simulink model "tractioncontrol_rmse22_nobrakes"  (R2022a)
settings: Solver=VariableStepAuto  StartTime=0.0  StopTime=48  RelTol=1e-3
values from neighbouring files (symbols this model uses):
  A = 1.08    [test_script.m]
  Cd = 1.02    [test_script.m]
  g = 9.81    [test_script.m]
  gr = 47/13    (= 3.61538461538)    [test_script.m]
  h_cg = .259    (= 0.259)    [test_script.m]
  h_d = h_cg    (= 0.259)    [test_script.m]
  J = 0.27    [test_script.m]
  m = 297    [test_script.m]
  r = 0.5588    [test_script.m]
  rho = 1.162    [test_script.m]
  wb = 1.53    [test_script.m]
undefined symbols (not defined in the file or in its folder): batt_Vnom, Conv_eff, front_wb, initial_SOC, motor_eff, normalized_voltage, Qmax, SOC
libraries: simulink x2, slpidlib x1
settings Model: Creator=Asus  LastModifiedBy=sahil
settings SolverCC: AlgebraicLoopSolver=TrustRegion
settings RTWCC: DLArmComputeVersion=19.05

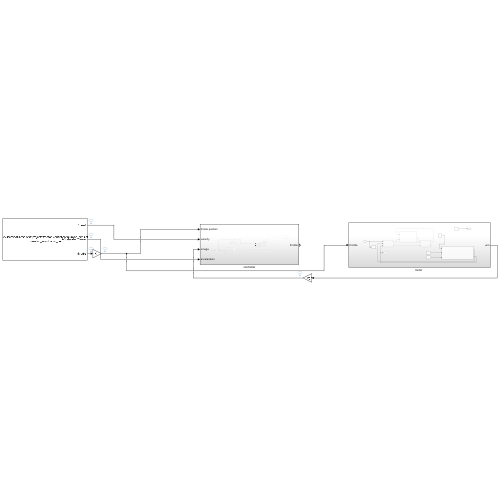
[thumbnail: Simulink's stored preview of the top-level diagram]
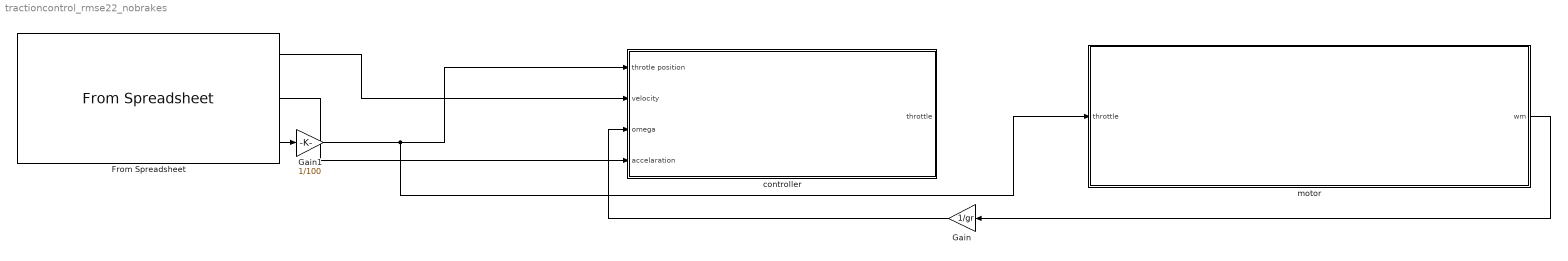
== system tractioncontrol_rmse22_nobrakes ==
  From Spreadsheet : FromSpreadsheet  FileName=C:\Users\sahil\rms stuff\projects\traction control\optimumlap_simulations\simulation_resultsssss_aaa.csv  SheetName=simulation_resultsssss_aaa
  Gain : Gain  Gain=1/gr
  Gain1 : Gain  Gain=1/100
  controller : Subsystem
  "motor  " : Subsystem
  wires:
  From Spreadsheet/3 -> Gain1/1
  "motor  "/1(wm) -> Gain/1
  Gain/1 -> controller/3(omega)
  From Spreadsheet/1 -> controller/2(velocity)
  From Spreadsheet/2 -> controller/4(accelaration)
  Gain1/1 -> "motor  "/1(throttle), controller/1(throtle position)

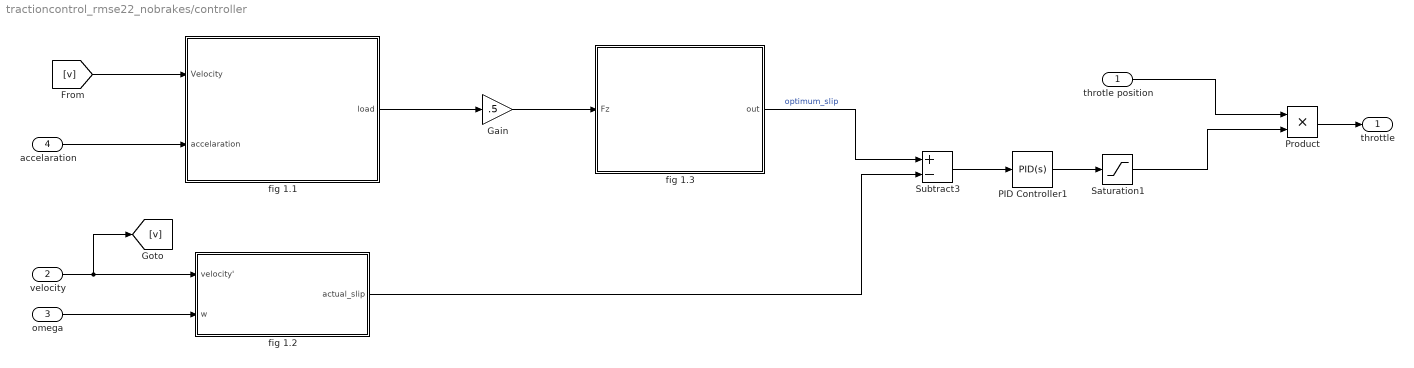
== system tractioncontrol_rmse22_nobrakes/controller ==
  throtle position : Inport
  velocity : Inport  Port=2
  omega : Inport  Port=3
  accelaration : Inport  Port=4
  Gain : Gain  Gain=.5
  PID Controller1 : slpidlib/PID Controller  Controller=PID  Form=Parallel  TimeDomain=Continuous-time  UseExternalTs=off  SampleTime=-1  IntegratorMethod=Forward Euler  FilterMethod=Forward Euler  ControllerParametersSource=internal  P=0.5  I=0.03  UseKiTs=off  D=0  N=100  UseFilter=on  TunerSelectOption=Transfer Function Based (PID Tuner App)  InitialConditionSource=internal  InitialConditionForIntegrator=0  InitialConditionForFilter=0  DifferentiatorICPrevScaledInput=0  ExternalReset=none  TrackingMode=off  Kt=1  LimitOutput=off  SatLimitsSource=internal  UpperSaturationLimit=inf  LowerSaturationLimit=-inf  LinearizeAsGain=on  AntiWindupMode=none  Kb=1  POutMin=[]  POutMax=[]  IOutMin=[]  IOutMax=[]  DOutMin=[]  DOutMax=[]  NOutMin=[]  NOutMax=[]  SumOutMin=[]  SumOutMax=[]  SaturationOutMin=[]  SaturationOutMax=[]  PParamMin=[]  PParamMax=[]  IParamMin=[]  IParamMax=[]  DParamMin=[]  DParamMax=[]  NParamMin=[]  NParamMax=[]  KbParamMin=[]  KbParamMax=[]  KtParamMin=[]  KtParamMax=[]  KbOutMin=[]  KbOutMax=[]  KtOutMin=[]  KtOutMax=[]  IntegratorOutMin=[]  IntegratorOutMax=[]  FilterOutMin=[]  FilterOutMax=[]  SumI1OutMin=[]  SumI1OutMax=[]  SumI2OutMin=[]  SumI2OutMax=[]  SumI3OutMin=[]  SumI3OutMax=[]  SumI4OutMin=[]  SumI4OutMax=[]  SumDOutMin=[]  SumDOutMax=[]  DifferentiatorOutMin=[]  DifferentiatorOutMax=[]  FilterDiffOutCoefMin=[]  FilterDiffOutCoefMax=[]  ReciprocalOutMin=[]  ReciprocalOutMax=[]  SumDenOutMin=[]  SumDenOutMax=[]  SumNumOutMin=[]  SumNumOutMax=[]  DivideOutMin=[]  DivideOutMax=[]  UdiffTsProdOutMin=[]  UdiffTsProdOutMax=[]  NTsProdOutMin=[]  NTsProdOutMax=[]  UintegralTsProdOutMin=[]  UintegralTsProdOutMax=[]  UngainTsProdOutMin=[]  UngainTsProdOutMax=[]  IntegratorContinuousStateAttributes=''  IntegratorStateMustResolveToSignalObject=off  IntegratorRTWStateStorageClass=Auto  FilterContinuousStateAttributes=''  FilterStateMustResolveToSignalObject=off  FilterRTWStateStorageClass=Auto  ParallelPVariant=InternalParameters  IdealPVariant=Disabled  IVariant=InternalParameters  DVariant=InternalParameters  IntegratorVariant=Continuous  SatVariant=Disabled  AWVariant=Passthrough  PCopyVariant=Disabled  TRVariant=Disabled  FdbkBlocksVariant=Forward  IdealPFdbkVariant=Disabled  SatFdbkVariant=Disabled  DerivativeFilterVariant=ContFilter  NVariant=InternalParameters  NCopyVariant=Disabled  FilterICVariant=InternalICsFilter  IntegratorICVariant=InternalICs  ExternalResetVariant=Disabled  TRSumVariant=Passthrough  SumFdbkVariant=Disabled  SumVariant=Sum_PID  TsampFilterVariant=InternalTs  TsampNgainVariant=Passthrough  TsampIntegralVariant=Passthrough  ExternalSaturationOutDataTypeStr=Inherit: Same as second input  aMode=0
  Product : Product
  Saturation1 : Saturate  UpperLimit=1  LowerLimit=-1
  Subtract3 : Sum  Inputs=+-
  fig 1.1 : Subsystem
  fig 1.2 : Subsystem
  fig 1.3 : MATLAB Function  TreatAsAtomicUnit=on
  throttle : Outport
  wires:
  Product/1 -> throttle/1
  fig 1.2/1(actual_slip) -> Subtract3/2
  Gain/1 -> fig 1.3/1(Fz)
  throtle position/1 -> Product/1
  fig 1.3/1(out) -> Subtract3/1  "optimum_slip"
  PID Controller1/1 -> Saturation1/1
  Subtract3/1 -> PID Controller1/1
  fig 1.1/1(load) -> Gain/1
  omega/1 -> fig 1.2/2(w)
  accelaration/1 -> fig 1.1/2(accelaration)
  velocity/1 -> [v], fig 1.2/1(velocity')
  [v] -> fig 1.1/1(Velocity)
  Saturation1/1 -> Product/2

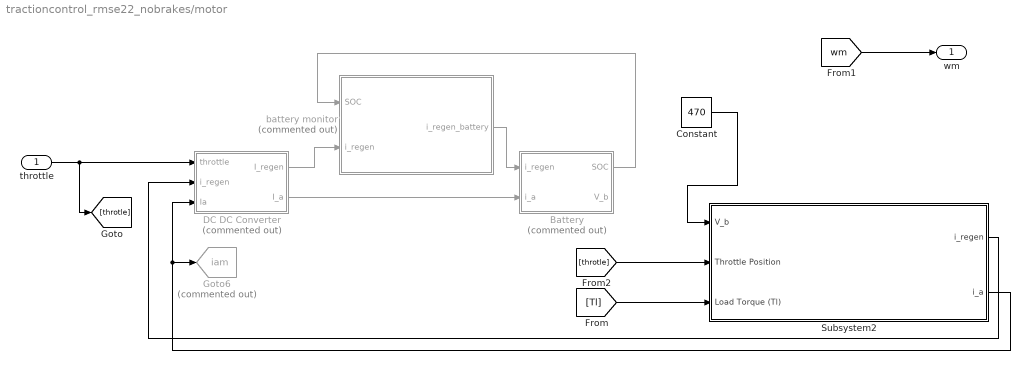
== system tractioncontrol_rmse22_nobrakes/motor   ==
  throttle : Inport
  Battery : Subsystem  Commented=on
  Constant : Constant  Value=470
  DC DC Converter : Subsystem  Commented=on
  Goto6 : Goto  Commented=on  GotoTag=iam  TagVisibility=global
  Subsystem2 : Subsystem
  battery monitor : Subsystem  Commented=on
  wm : Outport
  wires:
  Subsystem2/2(i_a) -> DC DC Converter/3(Ia), Goto6/1
  DC DC Converter/2(I_a) -> Battery/2(i_a)
  DC DC Converter/1(I_regen) -> battery monitor/2(i_regen)
  Subsystem2/1(i_regen) -> DC DC Converter/2(i_regen)
  throttle/1 -> [throtle], DC DC Converter/1(throttle)
  battery monitor/1(i_regen_battery) -> Battery/1(i_regen)
  Battery/1(SOC) -> battery monitor/1(SOC)
  [throtle] -> Subsystem2/2(Throttle Position)
  [Tl] -> Subsystem2/3(Load Torque (Tl))
  [wm] -> wm/1
  Constant/1 -> Subsystem2/1(V_b)

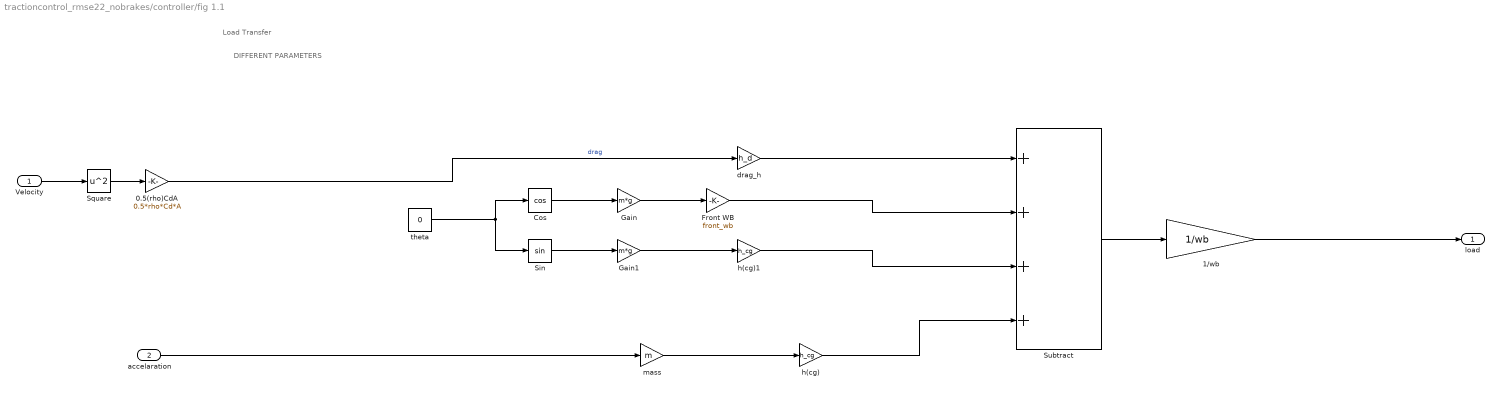
== system tractioncontrol_rmse22_nobrakes/controller/fig 1.1 ==
  note: Load Transfer
  note: DIFFERENT PARAMETERS
  Velocity : Inport
  accelaration : Inport  Port=2
  0.5(rho)CdA : Gain  Gain=0.5*rho*Cd*A
  1/wb : Gain  Gain=1/wb
  Cos : Trigonometry  Operator=cos
  Front WB : Gain  Gain=front_wb
  Gain : Gain  Gain=m*g
  Gain1 : Gain  Gain=m*g
  Sin : Trigonometry
  Square : Math  Operator=square
  Subtract : Sum  Inputs=++++
  drag_h : Gain  Gain=h_d
  h(cg) : Gain  Gain=h_cg
  h(cg)1 : Gain  Gain=h_cg
  mass : Gain  Gain=m
  theta : Constant  Value=0
  load : Outport
  wires:
  0.5(rho)CdA/1 -> drag_h/1  "drag"
  Velocity/1 -> Square/1
  1/wb/1 -> load/1
  Square/1 -> 0.5(rho)CdA/1
  Cos/1 -> Gain/1
  theta/1 -> Sin/1, Cos/1
  Sin/1 -> Gain1/1
  mass/1 -> h(cg)/1
  drag_h/1 -> Subtract/1
  Front WB/1 -> Subtract/2
  h(cg)1/1 -> Subtract/3
  h(cg)/1 -> Subtract/4
  Subtract/1 -> 1/wb/1
  accelaration/1 -> mass/1
  Gain/1 -> Front WB/1
  Gain1/1 -> h(cg)1/1

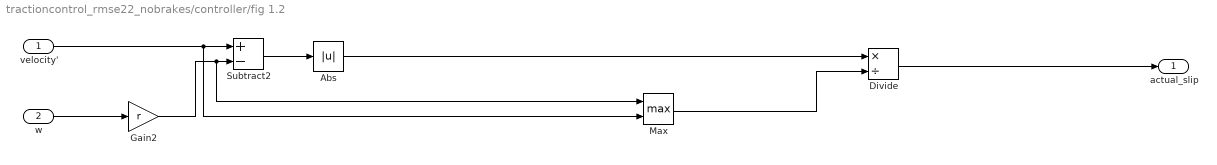
== system tractioncontrol_rmse22_nobrakes/controller/fig 1.2 ==
  velocity' : Inport
  w : Inport  Port=2
  Abs : Abs  SaturateOnIntegerOverflow=off
  Divide : Product  Inputs=*/
  Gain2 : Gain  Gain=r
  Max : MinMax  Function=max  Inputs=2
  Subtract2 : Sum  Inputs=+-
  actual_slip : Outport
  wires:
  Max/1 -> Divide/2
  velocity'/1 -> Max/2, Subtract2/1
  Gain2/1 -> Max/1, Subtract2/2
  w/1 -> Gain2/1
  Subtract2/1 -> Abs/1
  Abs/1 -> Divide/1
  Divide/1 -> actual_slip/1

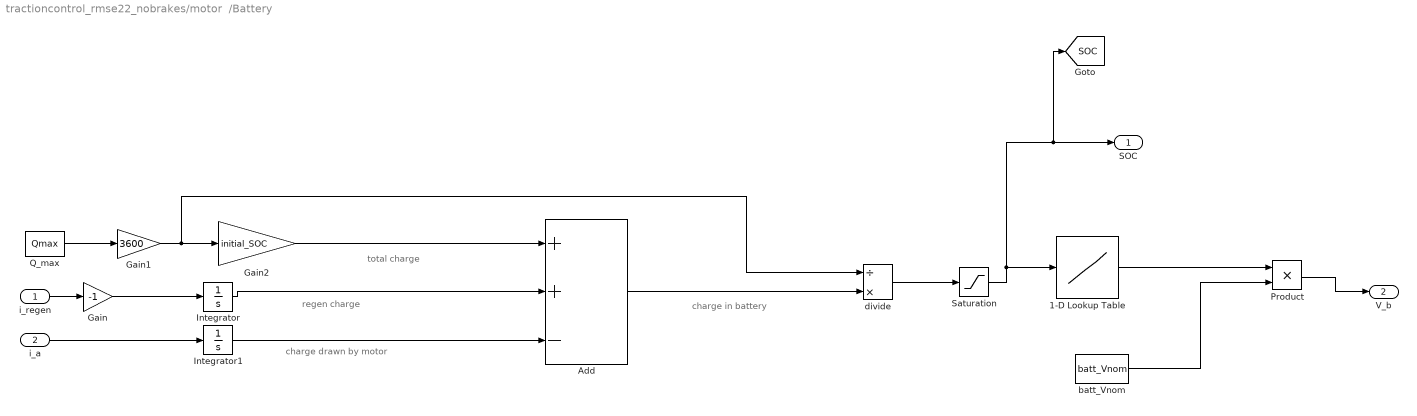
== system tractioncontrol_rmse22_nobrakes/motor  /Battery ==
  note: charge in battery
  note: total charge
  note: charge drawn by motor
  note: regen charge
  i_regen : Inport
  i_a : Inport  Port=2
  1-D Lookup Table : Lookup_n-D  NumberOfTableDimensions=1  BreakpointsForDimension1=SOC  Table=normalized_voltage  InternalRulePriority=Speed  RndMeth=Simplest
  Add : Sum  Inputs=++-
  Gain : Gain  Gain=-1
  Gain1 : Gain  Gain=3600
  Gain2 : Gain  Gain=initial_SOC
  Integrator : Integrator
  Integrator1 : Integrator
  Product : Product
  Q_max : Constant  Value=Qmax
  Saturation : Saturate  UpperLimit=1  LowerLimit=0
  batt_Vnom : Constant  Value=batt_Vnom
  divide : Product  Inputs=/*
  SOC : Outport
  V_b : Outport  Port=2
  tag scope: SOC=global
  wires:
  Integrator/1 -> Add/2
  i_a/1 -> Integrator1/1
  batt_Vnom/1 -> Product/2
  Gain/1 -> Integrator/1
  Gain2/1 -> Add/1
  Q_max/1 -> Gain1/1
  Gain1/1 -> divide/1, Gain2/1
  Add/1 -> divide/2
  i_regen/1 -> Gain/1
  Integrator1/1 -> Add/3
  Saturation/1 -> [SOC], SOC/1, 1-D Lookup Table/1
  1-D Lookup Table/1 -> Product/1
  divide/1 -> Saturation/1
  Product/1 -> V_b/1

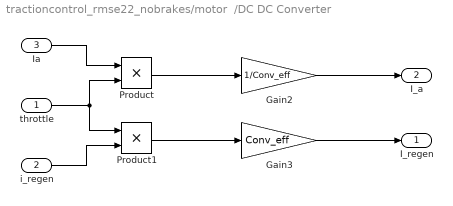
== system tractioncontrol_rmse22_nobrakes/motor  /DC DC Converter ==
  throttle : Inport
  i_regen : Inport  Port=2
  Ia : Inport  Port=3
  Gain2 : Gain  Gain=1/Conv_eff
  Gain3 : Gain  Gain=Conv_eff
  Product : Product
  Product1 : Product
  I_regen : Outport
  I_a : Outport  Port=2
  wires:
  Product1/1 -> Gain3/1
  throttle/1 -> Product/2, Product1/1
  Product/1 -> Gain2/1
  Gain3/1 -> I_regen/1
  Gain2/1 -> I_a/1
  Ia/1 -> Product/1
  i_regen/1 -> Product1/2

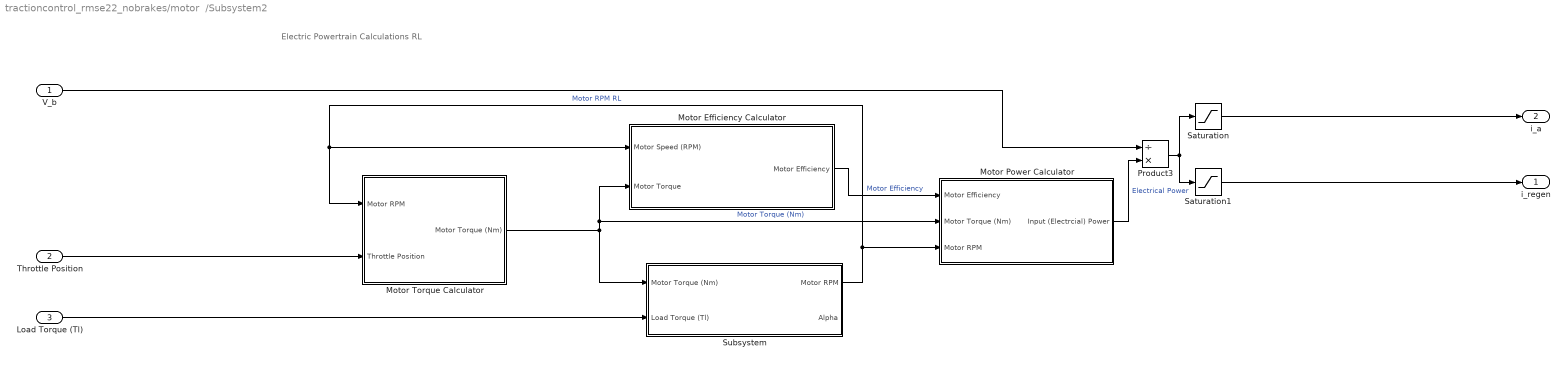
== system tractioncontrol_rmse22_nobrakes/motor  /Subsystem2 ==
  note: Electric Powertrain Calculations RL
  V_b : Inport
  Throttle Position : Inport  Port=2
  Load Torque (Tl) : Inport  Port=3
  Motor Efficiency Calculator : Subsystem
  Motor Power Calculator : Subsystem
  Motor Torque Calculator : Subsystem
  Product3 : Product  Inputs=/*
  Saturation : Saturate  UpperLimit=inf  LowerLimit=0
  Saturation1 : Saturate  UpperLimit=0  LowerLimit=-inf
  Subsystem : Subsystem
  i_regen : Outport
  i_a : Outport  Port=2
  wires:
  Motor Torque Calculator/1(Motor Torque (Nm)) -> Motor Efficiency Calculator/2(Motor Torque), Motor Power Calculator/2(Motor Torque (Nm)), Subsystem/1(Motor Torque (Nm))  "Motor Torque (Nm)"
  Product3/1 -> Saturation1/1, Saturation/1
  Motor Efficiency Calculator/1(Motor Efficiency) -> Motor Power Calculator/1(Motor Efficiency)  "Motor Efficiency"
  Motor Power Calculator/1(Input (Electrcial) Power) -> Product3/2  "Electrical Power"
  Subsystem/1(Motor RPM) -> Motor Torque Calculator/1(Motor RPM), Motor Efficiency Calculator/1(Motor Speed (RPM)), Motor Power Calculator/3(Motor RPM)  "Motor RPM RL"
  Saturation/1 -> i_a/1
  V_b/1 -> Product3/1
  Load Torque (Tl)/1 -> Subsystem/2(Load Torque (Tl))
  Throttle Position/1 -> Motor Torque Calculator/2(Throttle Position)
  Saturation1/1 -> i_regen/1

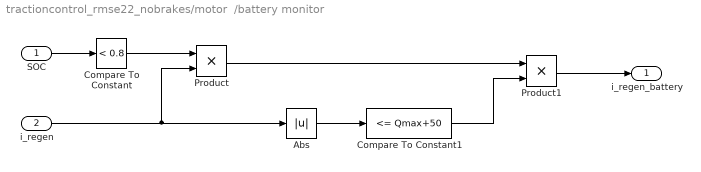
== system tractioncontrol_rmse22_nobrakes/motor  /battery monitor ==
  SOC : Inport
  i_regen : Inport  Port=2
  Abs : Abs  SaturateOnIntegerOverflow=off
  Compare To Constant : simulink/Logic and Bit Operations/Compare To Constant  relop=<  const=0.8  OutDataTypeStr=boolean
  Compare To Constant1 : simulink/Logic and Bit Operations/Compare To Constant  relop=<=  const=Qmax+50  OutDataTypeStr=boolean
  Product : Product
  Product1 : Product
  i_regen_battery : Outport
  wires:
  i_regen/1 -> Abs/1, Product/2
  SOC/1 -> Compare To Constant/1
  Compare To Constant/1 -> Product/1
  Abs/1 -> Compare To Constant1/1
  Product/1 -> Product1/1
  Compare To Constant1/1 -> Product1/2
  Product1/1 -> i_regen_battery/1

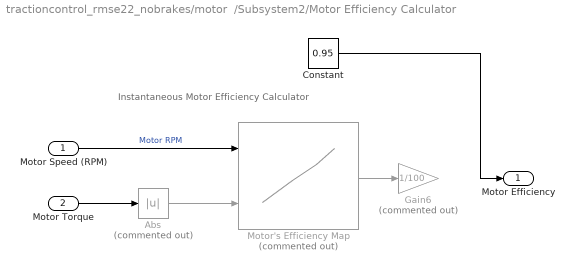
== system tractioncontrol_rmse22_nobrakes/motor  /Subsystem2/Motor Efficiency Calculator ==
  note: Instantaneous Motor Efficiency Calculator
  Motor Speed (RPM) : Inport
  Motor Torque : Inport  Port=2
  Abs : Abs  Commented=on  SaturateOnIntegerOverflow=off
  Constant : Constant  Value=0.95
  Gain6 : Gain  Commented=on  Gain=1/100
  Motor's Efficiency Map : Lookup_n-D  Commented=on  BreakpointsSpecification=Even spacing  BreakpointsForDimension1=|  BreakpointsForDimension2=[1:200]  BreakpointsForDimension1FirstPoint=0  BreakpointsForDimension2FirstPoint=0  BreakpointsForDimension1Spacing=500  BreakpointsForDimension2Spacing=50  Table=motor_eff  InternalRulePriority=Speed  RndMeth=Simplest
      | [10
      | 195
      | 398
      | 600
      | 795
      | 994
      | 1197
      | 1396
      | 1598
      | 1800
      | 1996
      | 2188
      | 2401
      | 2592
      | 2795
      | 2994
      | 3189
      | 3217
      | 3400
      | 3600
      | 3800
      | 4000
      | 4200
      | 4400
      | 4600
      | 4800
      | 5000
      | 5170
      | 5180]
      settings: InputPortMap=u0,u1
  Motor Efficiency : Outport
  wires:
  Motor's Efficiency Map/1 -> Gain6/1
  Motor Torque/1 -> Abs/1
  Motor Speed (RPM)/1 -> Motor's Efficiency Map/1  "Motor RPM"
  Abs/1 -> Motor's Efficiency Map/2
  Constant/1 -> Motor Efficiency/1

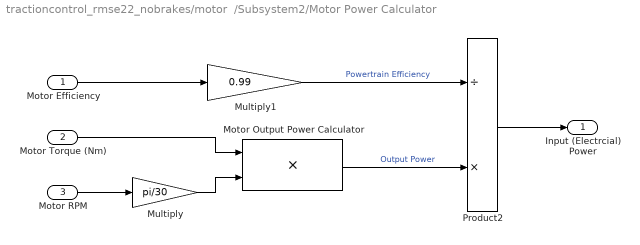
== system tractioncontrol_rmse22_nobrakes/motor  /Subsystem2/Motor Power Calculator ==
  Motor Efficiency : Inport
  Motor Torque (Nm) : Inport  Port=2
  Motor RPM : Inport  Port=3
  Motor Output Power Calculator : Product
  Multiply : Gain  Gain=pi/30
  Multiply1 : Gain  Gain=0.99
  Product2 : Product  Inputs=/*
  Input (Electrcial) Power : Outport
  wires:
  Product2/1 -> Input (Electrcial) Power/1
  Motor Output Power Calculator/1 -> Product2/2  "Output Power"
  Multiply/1 -> Motor Output Power Calculator/2
  Motor Torque (Nm)/1 -> Motor Output Power Calculator/1
  Multiply1/1 -> Product2/1  "Powertrain Efficiency"
  Motor Efficiency/1 -> Multiply1/1
  Motor RPM/1 -> Multiply/1

== system tractioncontrol_rmse22_nobrakes/motor  /Subsystem2/Motor Torque Calculator ==
  Motor RPM : Inport
  Throttle Position : Inport  Port=2
  Front motor characteristic curve2 : Lookup_n-D  NumberOfTableDimensions=1  BreakpointsForDimension1=[0 500 1000 1500 2000 2500 3183 3500 4000 4500 5000 5500 6000 6500 7000]  Table=[240 240 240 240 240 240 240 218.23 190.98 169.76 152.78 138.89 127.32 117.52 109.13]  InternalRulePriority=Speed  RndMeth=Simplest
  Product4 : Product
  Motor Torque (Nm) : Outport
  wires:
  Throttle Position/1 -> Product4/2
  Motor RPM/1 -> Front motor characteristic curve2/1
  Front motor characteristic curve2/1 -> Product4/1  "Max Available Torque (Nm)"
  Product4/1 -> Motor Torque (Nm)/1  "Motor Torque"

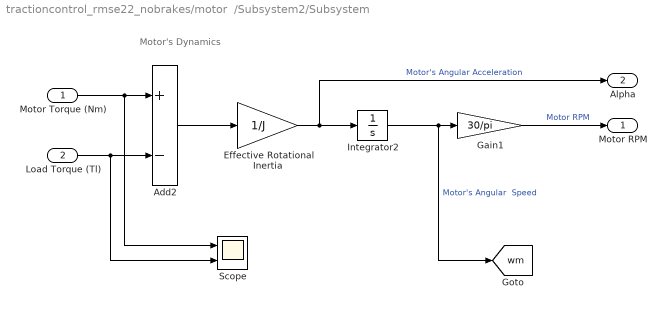
== system tractioncontrol_rmse22_nobrakes/motor  /Subsystem2/Subsystem ==
  note: Motor's Dynamics
  Motor Torque (Nm) : Inport
  Load Torque (Tl) : Inport  Port=2
  Add2 : Sum  Inputs=+-
  Effective Rotational Inertia : Gain  Gain=1/J
  Gain1 : Gain  Gain=30/pi
  Integrator2 : Integrator  InitialCondition=390
  Scope : Scope  NumInputPorts=2
  Motor RPM : Outport
  Alpha : Outport  Port=2
  tag scope: wm=global
  wires:
  Gain1/1 -> Motor RPM/1  "Motor RPM"
  Effective Rotational Inertia/1 -> Alpha/1, Integrator2/1  "Motor's Angular Acceleration"
  Add2/1 -> Effective Rotational Inertia/1
  Motor Torque (Nm)/1 -> Scope/1, Add2/1
  Load Torque (Tl)/1 -> Scope/2, Add2/2
  Integrator2/1 -> [wm], Gain1/1  "Motor's Angular  Speed"

== matlab function tractioncontrol_rmse22_nobrakes/controller/fig 1.3 ==
  data: Fz input; out output
function out  =packeja(Fz)
    
    a1=-2.13*(10^-5);
    a2=1.144;
    a3=4.96*(10^-5);
    a4=.226;
    a5=6.9*(10^-5);
    a6=-6*(10^-9);
    a7=5.6*(10*(-5));
    a8=.486;
    
    lambda=0:.005:1;
    Cx=1.65;
    Dx=a1*Fz*Fz+a2*Fz;
    func1=(a3*Fz*Fz+a4*Fz)*exp(-a5*Fz);
    Bx=func1/(Cx*Dx);
    Ex=a6*Fz*Fz+a7*Fz+a8;
    G=Bx*lambda;
    func2=G*(1-Ex)+Ex*atan(G);
    Fx=Dx*sin(Cx*atan(func2));
    plot(lambda,Fx)
    [~,I]=max(Fx);
    slip=lambda(I);
    out=slip;

end
